simulink model "total_2015a"  (R2015a)
settings: Solver=ode45  SolverMode=SingleTasking  StartTime=0.0  StopTime=10.0  RelTol=1e-3
values from neighbouring files (symbols this model uses):
  G = 9.8    [main.m]
  Kt = 3.575e-5    (= 3.575e-05)    [main.m]
  M = 1    [main.m]
  omega_0 = sqrt(G*M/Kt)    [main.m]
  u_0 = omega_0    [main.m]
  Z0 = 2    [main.m]
undefined symbols (not defined in the file or in its folder): i
settings Model: CovMetricSettings=dwe  CovHtmlReporting=off  covSaveCumulativeToWorkspaceVar=off  CovSaveSingleToWorkspaceVar=off  CovExternalEMLEnable=on  Creator=josem  LastModifiedBy=josem
settings DataIOCC: LimitDataPoints=off  SaveFormat=Dataset  ReturnWorkspaceOutputs=on
settings DebuggingCC: SFUnexpectedBacktrackingDiag=error  SFNoUnconditionalDefaultTransitionDiag=error
settings HardwareCC: ProdBitPerPointer=64  ProdLargestAtomicFloat=Float  ProdIntDivRoundTo=Zero  ProdEndianess=LittleEndian  ProdHWDeviceType=Specified
settings ModelReferenceCC: PropagateSignalLabelsOutOfModel=on
settings SFSimCC: SimUseLocalCustomCode=on
settings RTWCC: RTWUseLocalCustomCode=on
settings GRTTargetCC: TargetLangStandard=C99 (ISO)

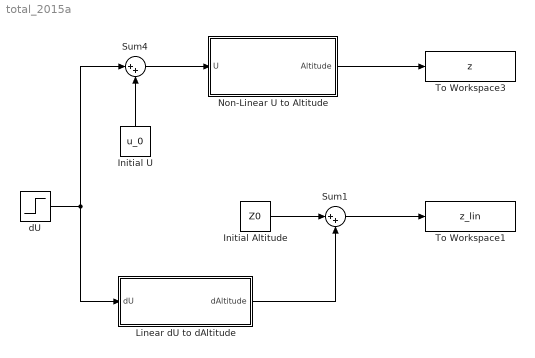
== system total_2015a ==
  Initial Altitude : Constant  Value=Z0
  Initial U : Constant  Value=u_0
  Linear dU to dAltitude : Subsystem
  Non-Linear U to Altitude : Subsystem
  Sum1 : Sum  Inputs=|++
  Sum4 : Sum  Inputs=|++
  To Workspace1 : ToWorkspace  VariableName=z_lin  SaveFormat=Structure With Time  SampleTime=-1
  To Workspace3 : ToWorkspace  VariableName=z  SaveFormat=Structure With Time  SampleTime=-1
  dU : Step  After=u(i)-u_0  SampleTime=0
  wires:
  Sum1/1 -> To Workspace1/1
  Initial Altitude/1 -> Sum1/1
  Initial U/1 -> Sum4/2
  dU/1 -> Linear dU to dAltitude/1(dU), Sum4/1
  Sum4/1 -> Non-Linear U to Altitude/1(U)
  Non-Linear U to Altitude/1(Altitude) -> To Workspace3/1
  Linear dU to dAltitude/1(dAltitude) -> Sum1/2

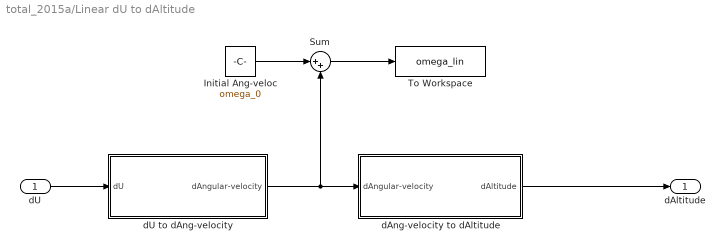
== system total_2015a/Linear dU to dAltitude ==
  dU : Inport
  Initial Ang-veloc : Constant  Value=omega_0
  Sum : Sum  Inputs=|++
  To Workspace : ToWorkspace  VariableName=omega_lin  SaveFormat=Structure With Time  SampleTime=-1
  dAng-velocity to dAltitude : Subsystem
  dU to dAng-velocity : Subsystem
  dAltitude : Outport
  wires:
  dAng-velocity to dAltitude/1(dAltitude) -> dAltitude/1
  dU to dAng-velocity/1(dAngular-velocity) -> dAng-velocity to dAltitude/1(dAngular-velocity), Sum/2
  dU/1 -> dU to dAng-velocity/1(dU)
  Initial Ang-veloc/1 -> Sum/1
  Sum/1 -> To Workspace/1

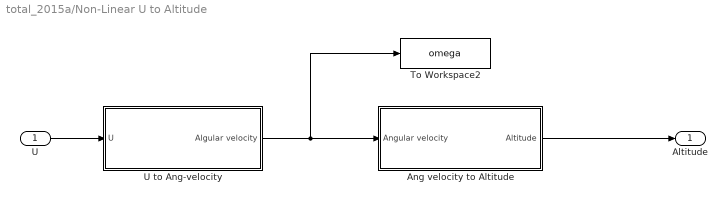
== system total_2015a/Non-Linear U to Altitude ==
  U : Inport
  Ang velocity to Altitude : Subsystem
  To Workspace2 : ToWorkspace  VariableName=omega  SaveFormat=Structure With Time  SampleTime=-1
  U to Ang-velocity : Subsystem
  Altitude : Outport
  wires:
  U to Ang-velocity/1(Algular velocity) -> To Workspace2/1, Ang velocity to Altitude/1(Angular velocity)
  Ang velocity to Altitude/1(Altitude) -> Altitude/1
  U/1 -> U to Ang-velocity/1(U)

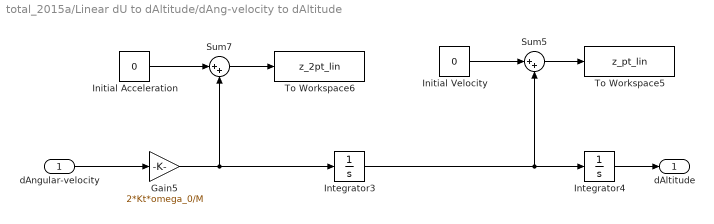
== system total_2015a/Linear dU to dAltitude/dAng-velocity to dAltitude ==
  dAngular-velocity : Inport
  Gain5 : Gain  Gain=2*Kt*omega_0/M
  Initial Acceleration : Constant  Value=0
  Initial Velocity : Constant  Value=0
  Integrator3 : Integrator
  Integrator4 : Integrator
  Sum5 : Sum  Inputs=|++
  Sum7 : Sum  Inputs=|++
  To Workspace5 : ToWorkspace  VariableName=z_pt_lin  SaveFormat=Structure With Time  SampleTime=-1
  To Workspace6 : ToWorkspace  VariableName=z_2pt_lin  SaveFormat=Structure With Time  SampleTime=-1
  dAltitude : Outport
  wires:
  Initial Velocity/1 -> Sum5/1
  Initial Acceleration/1 -> Sum7/1
  Integrator3/1 -> Integrator4/1, Sum5/2
  Sum5/1 -> To Workspace5/1
  Integrator4/1 -> dAltitude/1
  Sum7/1 -> To Workspace6/1
  Gain5/1 -> Integrator3/1, Sum7/2
  dAngular-velocity/1 -> Gain5/1

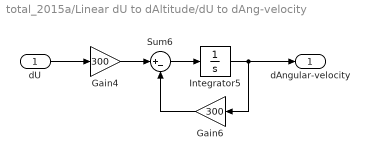
== system total_2015a/Linear dU to dAltitude/dU to dAng-velocity ==
  dU : Inport
  Gain4 : Gain  Gain=300
  Gain6 : Gain  Gain=300
  Integrator5 : Integrator
  Sum6 : Sum  Inputs=|+-
  dAngular-velocity : Outport
  wires:
  Gain4/1 -> Sum6/1
  Gain6/1 -> Sum6/2
  Integrator5/1 -> dAngular-velocity/1, Gain6/1
  Sum6/1 -> Integrator5/1
  dU/1 -> Gain4/1

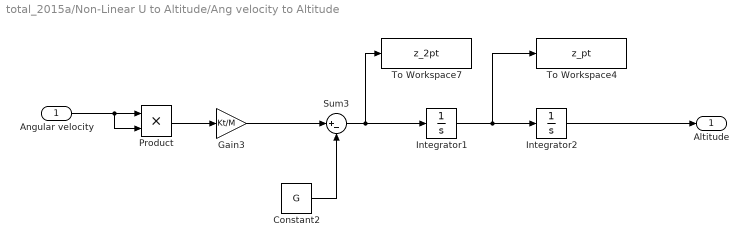
== system total_2015a/Non-Linear U to Altitude/Ang velocity to Altitude ==
  Angular velocity : Inport
  Constant2 : Constant  Value=G
  Gain3 : Gain  Gain=Kt/M
  Integrator1 : Integrator
  Integrator2 : Integrator  InitialCondition=Z0
  Product : Product
  Sum3 : Sum  Inputs=|+-
  To Workspace4 : ToWorkspace  VariableName=z_pt  SaveFormat=Structure With Time  SampleTime=-1
  To Workspace7 : ToWorkspace  VariableName=z_2pt  SaveFormat=Structure With Time  SampleTime=-1
  Altitude : Outport
  wires:
  Integrator1/1 -> To Workspace4/1, Integrator2/1
  Sum3/1 -> To Workspace7/1, Integrator1/1
  Gain3/1 -> Sum3/1
  Angular velocity/1 -> Product/2, Product/1
  Product/1 -> Gain3/1
  Constant2/1 -> Sum3/2
  Integrator2/1 -> Altitude/1

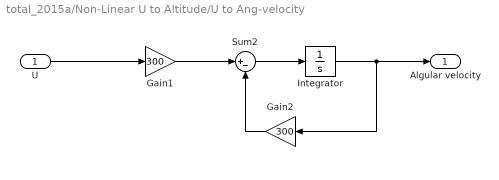
== system total_2015a/Non-Linear U to Altitude/U to Ang-velocity ==
  U : Inport
  Gain1 : Gain  Gain=300
  Gain2 : Gain  Gain=300
  Integrator : Integrator  InitialCondition=omega_0  LimitOutput=on  UpperSaturationLimit=3*omega_0  LowerSaturationLimit=0
  Sum2 : Sum  Inputs=|+-
  Algular velocity : Outport
  wires:
  Integrator/1 -> Algular velocity/1, Gain2/1
  Gain2/1 -> Sum2/2
  U/1 -> Gain1/1
  Gain1/1 -> Sum2/1
  Sum2/1 -> Integrator/1
